simulink model "testOpenLoopSim"  (R2016a)
settings: Solver=ode45  StartTime=0.0  StopTime=2  MaxStep=1e-4  RelTol=1e-6
values from neighbouring files (symbols this model uses):
  tStar = T(14e3: 10: 20e3) - T(14e3)    [runOrbitLinearization_backup.m]    (also in testOpenLoop.m = tStar{1})
  uStar = U(14e3: 10: 20e3)    [runOrbitLinearization_backup.m]    (also in testOpenLoop.m = uStar{1})
  x0 = Phi0(:,i)    [runOrbitLinearization_backup.m]    (also in testLinearEquilibrium.m = [0 0 0 0]'; testOpenLoop.m = [1 0 0 0]')
settings Model: Creator=xingye  LastModifiedBy=xingye

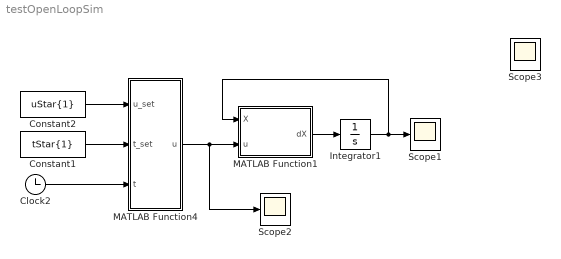
== system testOpenLoopSim ==
  Clock2 : Clock
  Constant1 : Constant  Value=tStar{1}
  Constant2 : Constant  Value=uStar{1}
  Integrator1 : Integrator  InitialCondition=x0
  MATLAB Function1 : MATLAB Function  TreatAsAtomicUnit=on
  MATLAB Function4 : MATLAB Function  TreatAsAtomicUnit=on
  Scope1 : Scope
  Scope2 : Scope
  Scope3 : Scope
  wires:
  MATLAB Function1/1(dX) -> Integrator1/1
  Integrator1/1 -> MATLAB Function1/1(X), Scope1/1
  MATLAB Function4/1(u) -> Scope2/1, MATLAB Function1/2(u)
  Clock2/1 -> MATLAB Function4/3(t)
  Constant2/1 -> MATLAB Function4/1(u_set)
  Constant1/1 -> MATLAB Function4/2(t_set)

== matlab function testOpenLoopSim/MATLAB Function1 ==
  data: X input size=4; u input size=1; dX output size=4
function dX = fcn(X, u)
%#codegen

% X = [0 pi/2 0 0]';
% u = 0;
%%
x = X(1:2);
x(2) = x(2) + pi/2;
xdot = X(3:4);

M = ([[2,-sin(x(2,:))/2];[-sin(x(2,:))/2,1/3]]);
f = ([[u(:,1)-xdot(1,:)/10+(xdot(2,:)^2*cos(x(2,:)))/2];[-xdot(2,:)/100-(981*cos(x(2,:)))/200]]);

xddot = M\f;

dX = [xdot; xddot];


% y = u;

== matlab function testOpenLoopSim/MATLAB Function4 ==
  data: u_set input; t_set input; u output; t input
function u = interp_u(u_set, t_set, t)
%#codegen

if sum(t_set) < 1
	u = 0;
else
	u = interp1(t_set', u_set', t,'spline');
end
